simulink model "Integrale_Estim"  (R2021a)
settings: Solver=FixedStepAuto  StartTime=0.0  StopTime=tf  FixedStep=Ts  RelTol=1e-3
undefined symbols (not defined in the file): a, N, Noise, P, Q, Ts
libraries: simulink x1
settings Model: Creator=perruquetti  LastModifiedBy=perruquetti

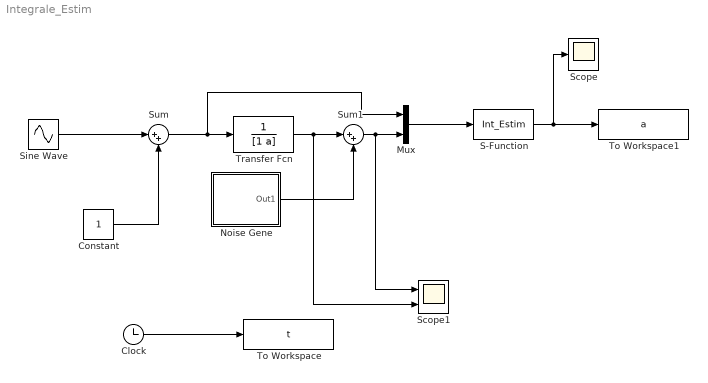
== system Integrale_Estim ==
  Clock : Clock
  Constant : Constant
  Mux : Mux  Inputs=2
  Noise Gene : Subsystem
  S-Function : S-Function  FunctionName=Int_Estim  Parameters=N,Ts,P,Q  SFunctionDeploymentMode=off  EnableBusSupport=off
  Scope : Scope
  Scope1 : Scope  NumInputPorts=2
  Sine Wave : Sin  Frequency=10  SampleTime=0
  Sum : Sum  Inputs=|++
  Sum1 : Sum  Inputs=|++
  To Workspace : ToWorkspace  VariableName=t  SampleTime=-1
  To Workspace1 : ToWorkspace  VariableName=a  SampleTime=-1
  Transfer Fcn : TransferFcn  Denominator=[1 a]  ParameterTunability=Unconstrained
  wires:
  Constant/1 -> Sum/2
  Sine Wave/1 -> Sum/1
  Sum/1 -> Mux/1, Transfer Fcn/1
  Clock/1 -> To Workspace/1
  Transfer Fcn/1 -> Sum1/1, Scope1/2
  Mux/1 -> S-Function/1
  S-Function/1 -> Scope/1, To Workspace1/1
  Noise Gene/1(Out1) -> Sum1/2
  Sum1/1 -> Scope1/1, Mux/2

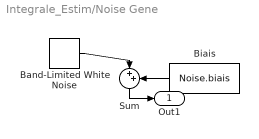
== system Integrale_Estim/Noise Gene ==
  Band-Limited White Noise : simulink/Sources/Band-Limited White Noise  Cov=Noise.power  Ts=Noise.sampling  seed=Noise.seed
  Biais : Constant  Value=Noise.biais
  Sum : Sum  Inputs=|++
  Out1 : Outport
  wires:
  Sum/1 -> Out1/1
  Biais/1 -> Sum/2
  Band-Limited White Noise/1 -> Sum/1
